simulink model "s0225"  (Simulink 6.0)
settings: Solver=ode3  SolverMode=SingleTasking  StartTime=0.0  StopTime=500  FixedStep=1  MaxStep=1  RelTol=1e-3  AbsTol=1e-6
values from neighbouring files (symbols this model uses):
  Kp = b01/a0*100    [m0221d.m]    (also in m0224.m = 3.3; m0225.m = 3.5; m0228.m = 1; m0232.m = 4)
  T1 = 3*T1    (= 0.3)    [m0203.m]    (also in m0204.m = 0.1; m0205.m = 0.1; m0207.m = 0.1; m0221d.m = 1/a0)
settings Model: LastModifiedBy=Froriep
settings DataIOCC: LimitDataPoints=off  SaveOutput=off  SaveTime=off
settings OptimizationCC: BooleanDataType=off
settings DebuggingCC: SolverPrmCheckMsg=none
settings HardwareCC: TargetUnknown=on
settings GRTTargetCC: ModelReferenceCompliant=off  MatFileLogging=off

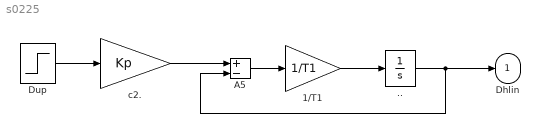
== system s0225 ==
  .. : Integrator  InitialCondition=1.e-6
  1/T1 : Gain  Gain=1/T1  SaturateOnIntegerOverflow=on
  A5 : Sum  Inputs=+-  SaturateOnIntegerOverflow=on  InputSameDT=on
  Dup : Step  Time=.1  SampleTime=0
  c2. : Gain  Gain=Kp  SaturateOnIntegerOverflow=on
  Dhlin : Outport
  wires:
  ../1 -> A5/2, Dhlin/1
  1/T1/1 -> ../1
  A5/1 -> 1/T1/1
  Dup/1 -> c2./1
  c2./1 -> A5/1
